simulink model "yenimodel"  (R2017b)
settings: Solver=VariableStepAuto  StartTime=0.0  StopTime=10.0  RelTol=1e-3
model workspace (MAT data in the model file):
  wc = 0
  wo = 0
undefined symbols (not defined in the file or in its folder): kiV, kpV, Ts_Power
libraries: powerlib x24, powerlib_meascontrol x4, re_lib x2, simulink x1
settings Model: Creator=ongun  LastModifiedBy=ongun

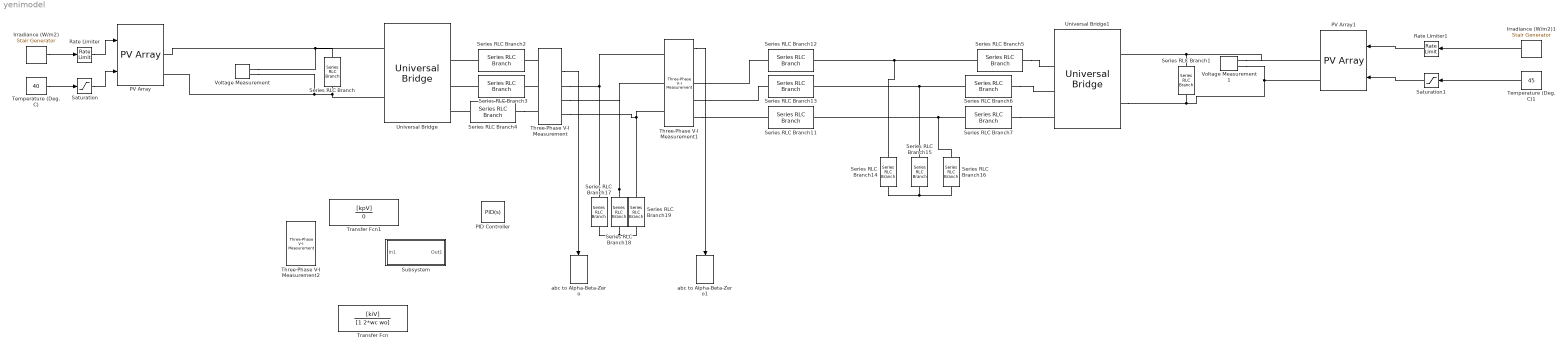
== system yenimodel ==
  Irradiance (W/m2) : powerlib_meascontrol/Pulse & Signal Generators/Stair Generator  t=[0, 0.4, 1.0]  e=[1, 0.2, 1]*1000  Ts=Ts_Power
      settings: SourceProductName=Simscape Power Systems
  Irradiance (W/m2)1 : powerlib_meascontrol/Pulse & Signal Generators/Stair Generator  t=[0, 0.4, 1.0]  e=[1, 0.2, 1]*1000  Ts=Ts_Power
      settings: SourceProductName=Simscape Power Systems
  PID Controller : simulink/Continuous/PID Controller  Controller=PID  TimeDomain=Continuous-time  SampleTime=-1  IntegratorMethod=Forward Euler  FilterMethod=Forward Euler  Form=Parallel  UseFilter=on  ControllerParametersSource=internal  P=1  I=1  D=0  N=100  InitialConditionSource=internal  InitialConditionForIntegrator=0  InitialConditionForFilter=0  ExternalReset=none  LimitOutput=off  UpperSaturationLimit=inf  LowerSaturationLimit=-inf  LinearizeAsGain=on  AntiWindupMode=none  Kb=1  TrackingMode=off  Kt=1  PParamMin=[]  PParamMax=[]  IParamMin=[]  IParamMax=[]  DParamMin=[]  DParamMax=[]  NParamMin=[]  NParamMax=[]  KbParamMin=[]  KbParamMax=[]  KtParamMin=[]  KtParamMax=[]  POutMin=[]  POutMax=[]  IOutMin=[]  IOutMax=[]  DOutMin=[]  DOutMax=[]  NOutMin=[]  NOutMax=[]  KbOutMin=[]  KbOutMax=[]  KtOutMin=[]  KtOutMax=[]  IntegratorOutMin=[]  IntegratorOutMax=[]  FilterOutMin=[]  FilterOutMax=[]  SumOutMin=[]  SumOutMax=[]  SumI1OutMin=[]  SumI1OutMax=[]  SumI2OutMin=[]  SumI2OutMax=[]  SumI3OutMin=[]  SumI3OutMax=[]  SumDOutMin=[]  SumDOutMax=[]  SaturationOutMin=[]  SaturationOutMax=[]  IntegratorContinuousStateAttributes=''  IntegratorStateMustResolveToSignalObject=off  IntegratorRTWStateStorageClass=Auto  FilterContinuousStateAttributes=''  FilterStateMustResolveToSignalObject=off  FilterRTWStateStorageClass=Auto  DifferentiatorICPrevScaledInput=0  DifferentiatorOutMin=[]  DifferentiatorOutMax=[]  InitialConditionSetting=State (most efficient)  FilterDiffOutCoefMin=[]  FilterDiffOutCoefMax=[]  SumDenOutMin=[]  SumDenOutMax=[]  SumNumOutMin=[]  SumNumOutMax=[]  ReciprocalOutMin=[]  ReciprocalOutMax=[]  DivideOutMin=[]  DivideOutMax=[]  TunerSelectOption=Transfer Function Based (PID Tuner App)
  PV Array : re_lib/Solar/PV Array  Npar=88  Nser=7  PlotType=array @ 1000 W/m2 & specified temperatures  S_vec="[ 1000  500  100 ]"  Temp_C_vec="[ 45 25  ]"  ModuleName=SunPower SPR-415E-WHT-D  PlotWhenSelected=off  Pm=414.801  Ncell=128  Voc=85.3  Isc=6.09  Vm=72.9  Im=5.69  beta_Voc_pc=-0.229  alpha_Isc_pc=0.030706  beta_Voc=-0.19534  alpha_Isc=0.00187  IL=6.0978  I0=7.1712e-13  nI=0.87223  Rsh=419.7813  Rs=0.5371  BAL=on  Tc=1e-6  Tfilter=5e-5
      settings: AttributesFormatString=|
      | %<ModuleName>
      | %<Nser>-module string
      | %<Npar> parallel strings
  PV Array1 : re_lib/Solar/PV Array  Npar=88  Nser=7  PlotType=array @ 1000 W/m2 & specified temperatures  S_vec="[ 1000  500  100 ]"  Temp_C_vec="[ 45 25  ]"  ModuleName=SunPower SPR-415E-WHT-D  PlotWhenSelected=off  Pm=414.801  Ncell=128  Voc=85.3  Isc=6.09  Vm=72.9  Im=5.69  beta_Voc_pc=-0.229  alpha_Isc_pc=0.030706  beta_Voc=-0.19534  alpha_Isc=0.00187  IL=6.0978  I0=7.1712e-13  nI=0.87223  Rsh=419.7813  Rs=0.5371  BAL=on  Tc=1e-6  Tfilter=5e-5
      settings: AttributesFormatString=|
      | %<ModuleName>
      | %<Nser>-module string
      | %<Npar> parallel strings
  Rate Limiter : RateLimiter  RisingSlewLimit=6000  FallingSlewLimit=-6000  SampleTimeMode=inherited  InitialCondition=1000
  Rate Limiter1 : RateLimiter  RisingSlewLimit=6000  FallingSlewLimit=-6000  SampleTimeMode=inherited  InitialCondition=1000
  Saturation : Saturate  UpperLimit=55  LowerLimit=5
  Saturation1 : Saturate  UpperLimit=55  LowerLimit=5
  Series RLC Branch{,1,14..19} (8 alike) : powerlib/Elements/Series RLC Branch  LConnTagsString=__new0  RConnTagsString=__new0  BranchType=C  Resistance=1  Inductance=1e-3  SetiL0=off  InitialCurrent=0  Capacitance=1e-6  Setx0=off  InitialVoltage=0  Measurements=None
  Series RLC Branch{2..7,11..13} (9 alike) : powerlib/Elements/Series RLC Branch  LConnTagsString=__new0  RConnTagsString=__new0  BranchType=L  Resistance=1  Inductance=1e-3  SetiL0=off  InitialCurrent=0  Capacitance=1e-6  Setx0=off  InitialVoltage=0  Measurements=None
  Subsystem : Subsystem
  Temperature (Deg. C) : Constant  Value=40
  Temperature (Deg. C)1 : Constant  Value=45
  Three-Phase V-I Measurement : powerlib/Measurements/Three-Phase V-I Measurement  VoltageMeasurement=phase-to-ground  SetLabelV=off  LabelV=Vabc  Vpu=off  VpuLL=off  CurrentMeasurement=yes  SetLabelI=off  LabelI=Iabc  Ipu=off  Pbase=100e6  Vbase=500e3  OutputType=Complex  PhasorSimulation=off  PSBequivalent=0
  Three-Phase V-I Measurement1 : powerlib/Measurements/Three-Phase V-I Measurement  VoltageMeasurement=phase-to-ground  SetLabelV=off  LabelV=Vabc  Vpu=off  VpuLL=off  CurrentMeasurement=yes  SetLabelI=off  LabelI=Iabc  Ipu=off  Pbase=100e6  Vbase=500e3  OutputType=Complex  PhasorSimulation=off  PSBequivalent=0
  Three-Phase V-I Measurement2 : powerlib/Measurements/Three-Phase V-I Measurement  VoltageMeasurement=phase-to-ground  SetLabelV=off  LabelV=Vabc  Vpu=off  VpuLL=off  CurrentMeasurement=yes  SetLabelI=off  LabelI=Iabc  Ipu=off  Pbase=100e6  Vbase=500e3  OutputType=Complex  PhasorSimulation=off  PSBequivalent=0
  Transfer Fcn : TransferFcn  Numerator=[kiV]  Denominator=[1 2*wc wo]
  Transfer Fcn1 : TransferFcn  Numerator=[kpV]  Denominator=[0 0 0]
  Universal Bridge : powerlib/Power Electronics/Universal Bridge  Arms=3  SnubberResistance=1e5  SnubberCapacitance=inf  Device=IGBT / Diodes  Ron=1e-3  Lon=0  ForwardVoltages="[  0  0  ]"  ForwardVoltage=0  GTOparameters=[ 10e-6 , 20e-6 ]  IGBTparameters=[ 1e-6 , 2e-6 ]  Measurements=None  Measurements_2=None  converterType=Rectifier
  Universal Bridge1 : powerlib/Power Electronics/Universal Bridge  Arms=3  SnubberResistance=1e5  SnubberCapacitance=inf  Device=IGBT / Diodes  Ron=1e-3  Lon=0  ForwardVoltages="[  0  0  ]"  ForwardVoltage=0  GTOparameters=[ 10e-6 , 20e-6 ]  IGBTparameters=[ 1e-6 , 2e-6 ]  Measurements=None  Measurements_2=None  converterType=Rectifier
  Voltage Measurement : powerlib/Measurements/Voltage Measurement  PhasorSimulation=off  OutputType=Complex  PSBequivalent=0
  Voltage Measurement1 : powerlib/Measurements/Voltage Measurement  PhasorSimulation=off  OutputType=Complex  PSBequivalent=0
  abc to Alpha-Beta-Zero : powerlib_meascontrol/Transformations/abc to Alpha-Beta-Zero
      settings: SourceProductName=Simscape Power Systems
  abc to Alpha-Beta-Zero1 : powerlib_meascontrol/Transformations/abc to Alpha-Beta-Zero
      settings: SourceProductName=Simscape Power Systems
  wires:
  Temperature (Deg. C)/1 -> Saturation/1
  Rate Limiter/1 -> PV Array/1
  Temperature (Deg. C)1/1 -> Saturation1/1
  Irradiance (W/m2)1/1 -> Rate Limiter1/1
  Saturation/1 -> PV Array/2
  Saturation1/1 -> PV Array1/2
  Rate Limiter1/1 -> PV Array1/1
  Irradiance (W/m2)/1 -> Rate Limiter/1
  Three-Phase V-I Measurement/2 -> abc to Alpha-Beta-Zero/1
  Three-Phase V-I Measurement1/1 -> abc to Alpha-Beta-Zero1/1
  connections:
  Universal Bridge/RConn2 -- Voltage Measurement/LConn2 -- PV Array/RConn2 -- Series RLC Branch/LConn1
  Voltage Measurement/LConn1 -- Series RLC Branch/RConn1 -- Universal Bridge/RConn1 -- PV Array/RConn1
  Series RLC Branch1/RConn1 -- PV Array1/RConn1 -- Voltage Measurement1/LConn1 -- Universal Bridge1/RConn1
  Universal Bridge1/RConn2 -- Voltage Measurement1/LConn2 -- PV Array1/RConn2 -- Series RLC Branch1/LConn1
  Series RLC Branch5/LConn1 -- Series RLC Branch14/RConn1 -- Series RLC Branch12/RConn1
  Series RLC Branch6/LConn1 -- Series RLC Branch15/RConn1 -- Series RLC Branch13/RConn1
  Series RLC Branch7/LConn1 -- Series RLC Branch16/RConn1 -- Series RLC Branch11/RConn1
  Series RLC Branch7/RConn1 -- Universal Bridge1/LConn3
  Series RLC Branch6/RConn1 -- Universal Bridge1/LConn2
  Series RLC Branch5/RConn1 -- Universal Bridge1/LConn1
  Series RLC Branch17/RConn1 -- Three-Phase V-I Measurement1/LConn1 -- Three-Phase V-I Measurement/RConn1
  Series RLC Branch2/LConn1 -- Universal Bridge/LConn1
  Series RLC Branch3/LConn1 -- Universal Bridge/LConn2
  Series RLC Branch18/RConn1 -- Three-Phase V-I Measurement1/LConn2 -- Three-Phase V-I Measurement/RConn2
  Three-Phase V-I Measurement/RConn3 -- Three-Phase V-I Measurement1/LConn3 -- Series RLC Branch19/RConn1
  Series RLC Branch4/LConn1 -- Universal Bridge/LConn3
  Series RLC Branch12/LConn1 -- Three-Phase V-I Measurement1/RConn1
  Three-Phase V-I Measurement1/RConn3 -- Series RLC Branch11/LConn1
  Series RLC Branch14/LConn1 -- Series RLC Branch15/LConn1 -- Series RLC Branch16/LConn1
  Series RLC Branch17/LConn1 -- Series RLC Branch19/LConn1 -- Series RLC Branch18/LConn1
  Three-Phase V-I Measurement/LConn1 -- Series RLC Branch2/RConn1
  Three-Phase V-I Measurement/LConn2 -- Series RLC Branch3/RConn1
  Series RLC Branch4/RConn1 -- Three-Phase V-I Measurement/LConn3
  Series RLC Branch13/LConn1 -- Three-Phase V-I Measurement1/RConn2

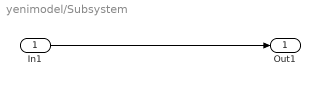
== system yenimodel/Subsystem ==
  In1 : Inport
  Out1 : Outport
  wires:
  In1/1 -> Out1/1
